simulink model "tanks_model"  (R2014a)
settings: Solver=ode4  StartTime=0.0  StopTime=T  FixedStep=0.001  RelTol=1e-3
values from neighbouring files (symbols this model uses):
  a = 31    [tanks_runner.m]
  b = 40    [tanks_runner.m]
  c = 10    [tanks_runner.m]
  C1 = 20    [tanks_runner.m]
  C2 = 20    [tanks_runner.m]
  C3 = 20    [tanks_runner.m]
  h10 = 13    [tanks_runner.m]
  h20 = 13    [tanks_runner.m]
  h30 = 7    [tanks_runner.m]
  h_max = 40    [tanks_runner.m]
  R = 40    [tanks_runner.m]
  u_max = 50    [tanks_runner.m]
  w = 5    [tanks_runner.m]
settings Model: Creator=Lukasz  LastModifiedBy=Lukasz

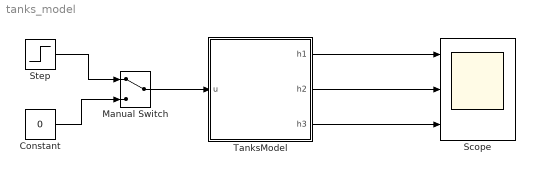
== system tanks_model ==
  Constant : Constant  Value=0
  Manual Switch : ManualSwitch
  Scope : Scope  NumInputPorts=3
      settings: ShowLegends=on  YMin=-0~-5~-5  YMax=40~5~5  SampleInput=on
  Step : Step  Time=0  After=u_max  SampleTime=0
  TanksModel : Subsystem
  wires:
  TanksModel/1(h1) -> Scope/1
  TanksModel/2(h2) -> Scope/2
  TanksModel/3(h3) -> Scope/3
  Manual Switch/1 -> TanksModel/1(u)
  Constant/1 -> Manual Switch/2
  Step/1 -> Manual Switch/1

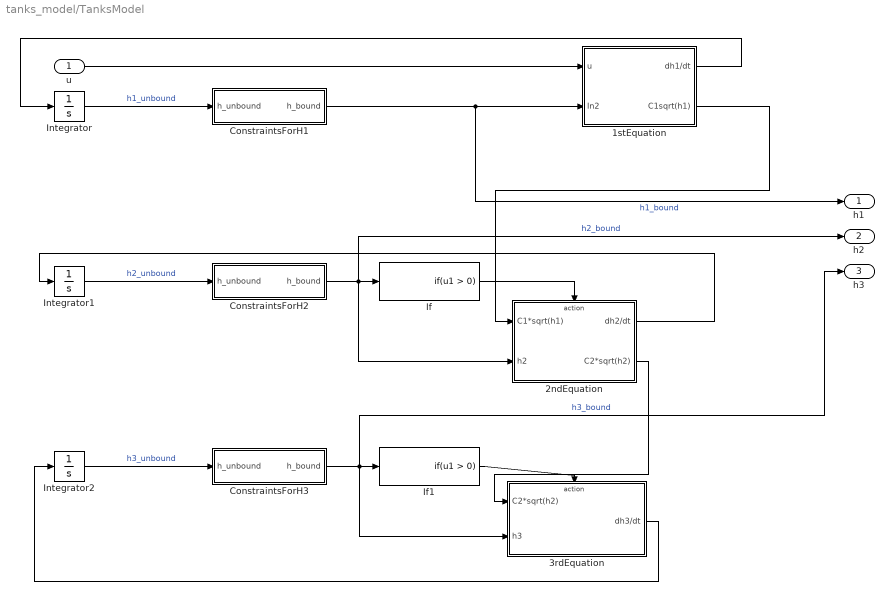
== system tanks_model/TanksModel ==
  u : Inport
  1stEquation : Subsystem
  2ndEquation : Subsystem
  3rdEquation : Subsystem
  ConstraintsForH1 : Subsystem
  ConstraintsForH2 : Subsystem
  ConstraintsForH3 : Subsystem
  If : If  ShowElse=off
  If1 : If  ShowElse=off
  Integrator : Integrator  InitialCondition=h10
  Integrator1 : Integrator  InitialCondition=h20
  Integrator2 : Integrator  InitialCondition=h30
  h1 : Outport
  h2 : Outport  Port=2
  h3 : Outport  Port=3
  wires:
  Integrator1/1 -> ConstraintsForH2/1(h_unbound)  "h2_unbound"
  Integrator2/1 -> ConstraintsForH3/1(h_unbound)  "h3_unbound"
  ConstraintsForH1/1(h_bound) -> h1/1, 1stEquation/2(In2)  "h1_bound"
  Integrator/1 -> ConstraintsForH1/1(h_unbound)  "h1_unbound"
  ConstraintsForH2/1(h_bound) -> If/1, 2ndEquation/2(h2), h2/1  "h2_bound"
  ConstraintsForH3/1(h_bound) -> If1/1, 3rdEquation/2(h3), h3/1  "h3_bound"
  2ndEquation/1(dh2/dt) -> Integrator1/1
  If/1 -> 2ndEquation/Action
  2ndEquation/2(C2*sqrt(h2)) -> 3rdEquation/1(C2*sqrt(h2))
  If1/1 -> 3rdEquation/Action
  3rdEquation/1(dh3/dt) -> Integrator2/1
  u/1 -> 1stEquation/1(u)
  1stEquation/1(dh1/dt) -> Integrator/1
  1stEquation/2(C1sqrt(h1)) -> 2ndEquation/1(C1*sqrt(h1))

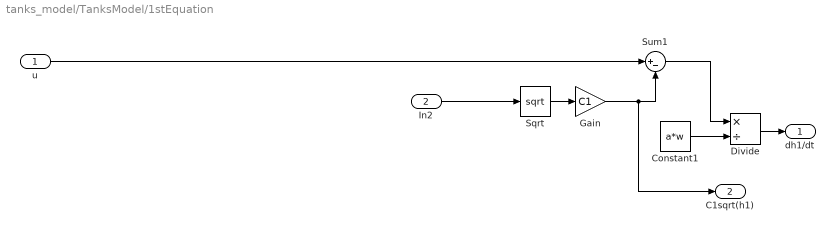
== system tanks_model/TanksModel/1stEquation ==
  u : Inport
  In2 : Inport  Port=2
  Constant1 : Constant  Value=a*w
  Divide : Product  Inputs=*/
  Gain : Gain  Gain=C1
  Sqrt : Sqrt  SaturateOnIntegerOverflow=on
  Sum1 : Sum  Inputs=|+-
  dh1/dt : Outport
  C1sqrt(h1) : Outport  Port=2
  wires:
  In2/1 -> Sqrt/1
  Constant1/1 -> Divide/2
  Divide/1 -> dh1/dt/1
  u/1 -> Sum1/1
  Gain/1 -> C1sqrt(h1)/1, Sum1/2
  Sqrt/1 -> Gain/1
  Sum1/1 -> Divide/1

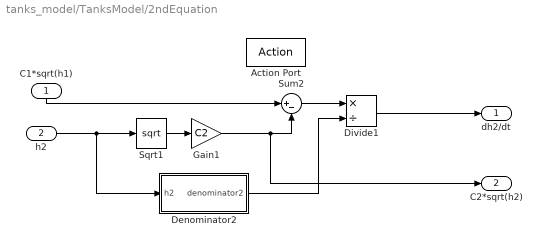
== system tanks_model/TanksModel/2ndEquation ==
  C1*sqrt(h1) : Inport
  h2 : Inport  Port=2
  Action Port : ActionPort  ActionType=then
  Denominator2 : Subsystem
  Divide1 : Product  Inputs=*/
  Gain1 : Gain  Gain=C2
  Sqrt1 : Sqrt  SaturateOnIntegerOverflow=on
  Sum2 : Sum  Inputs=|+-
  dh2/dt : Outport
  C2*sqrt(h2) : Outport  Port=2
  wires:
  Sqrt1/1 -> Gain1/1
  Gain1/1 -> C2*sqrt(h2)/1, Sum2/2
  Denominator2/1(denominator2) -> Divide1/2
  Sum2/1 -> Divide1/1
  Divide1/1 -> dh2/dt/1
  h2/1 -> Denominator2/1(h2), Sqrt1/1
  C1*sqrt(h1)/1 -> Sum2/1

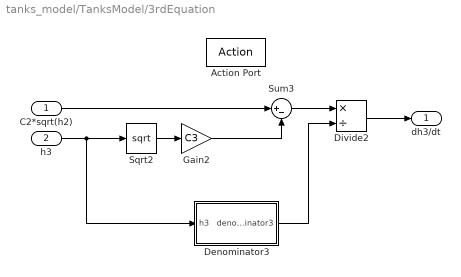
== system tanks_model/TanksModel/3rdEquation ==
  C2*sqrt(h2) : Inport
  h3 : Inport  Port=2
  Action Port : ActionPort  ActionType=then
  Denominator3 : Subsystem
  Divide2 : Product  Inputs=*/
  Gain2 : Gain  Gain=C3
  Sqrt2 : Sqrt  SaturateOnIntegerOverflow=on
  Sum3 : Sum  Inputs=|+-
  dh3/dt : Outport
  wires:
  Sum3/1 -> Divide2/1
  Divide2/1 -> dh3/dt/1
  Sqrt2/1 -> Gain2/1
  Gain2/1 -> Sum3/2
  Denominator3/1(denominator3) -> Divide2/2
  C2*sqrt(h2)/1 -> Sum3/1
  h3/1 -> Denominator3/1(h3), Sqrt2/1

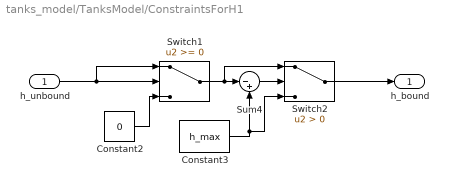
== system tanks_model/TanksModel/ConstraintsForH1 ==
  h_unbound : Inport
  Constant2 : Constant  Value=0
  Constant3 : Constant  Value=h_max
  Sum4 : Sum  Inputs=|-+
  Switch1 : Switch
  Switch2 : Switch  Criteria=u2 > Threshold
  h_bound : Outport
  wires:
  h_unbound/1 -> Switch1/2, Switch1/1
  Constant2/1 -> Switch1/3
  Switch1/1 -> Switch2/1, Sum4/1
  Switch2/1 -> h_bound/1
  Sum4/1 -> Switch2/2
  Constant3/1 -> Sum4/2, Switch2/3

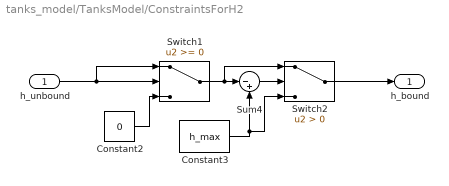
== system tanks_model/TanksModel/ConstraintsForH2 ==
  h_unbound : Inport
  Constant2 : Constant  Value=0
  Constant3 : Constant  Value=h_max
  Sum4 : Sum  Inputs=|-+
  Switch1 : Switch
  Switch2 : Switch  Criteria=u2 > Threshold
  h_bound : Outport
  wires:
  Constant3/1 -> Switch2/3, Sum4/2
  Sum4/1 -> Switch2/2
  Switch2/1 -> h_bound/1
  Switch1/1 -> Sum4/1, Switch2/1
  Constant2/1 -> Switch1/3
  h_unbound/1 -> Switch1/1, Switch1/2

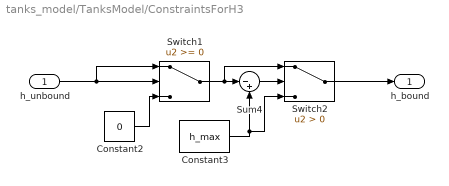
== system tanks_model/TanksModel/ConstraintsForH3 ==
  h_unbound : Inport
  Constant2 : Constant  Value=0
  Constant3 : Constant  Value=h_max
  Sum4 : Sum  Inputs=|-+
  Switch1 : Switch
  Switch2 : Switch  Criteria=u2 > Threshold
  h_bound : Outport
  wires:
  h_unbound/1 -> Switch1/2, Switch1/1
  Constant2/1 -> Switch1/3
  Switch1/1 -> Switch2/1, Sum4/1
  Switch2/1 -> h_bound/1
  Sum4/1 -> Switch2/2
  Constant3/1 -> Sum4/2, Switch2/3

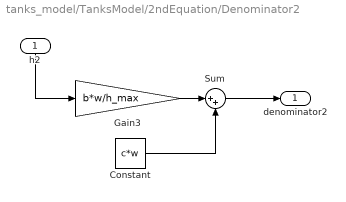
== system tanks_model/TanksModel/2ndEquation/Denominator2 ==
  h2 : Inport
  Constant : Constant  Value=c*w
  Gain3 : Gain  Gain=b*w/h_max
  Sum : Sum  Inputs=|++
  denominator2 : Outport
  wires:
  Sum/1 -> denominator2/1
  Constant/1 -> Sum/2
  h2/1 -> Gain3/1
  Gain3/1 -> Sum/1

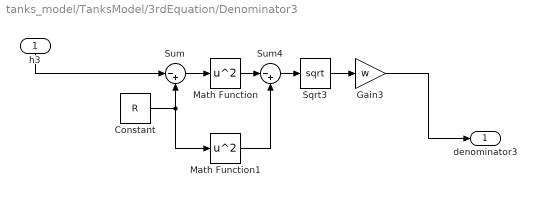
== system tanks_model/TanksModel/3rdEquation/Denominator3 ==
  h3 : Inport
  Constant : Constant  Value=R
  Gain3 : Gain  Gain=w
  Math Function : Math  Operator=square  SaturateOnIntegerOverflow=on
  Math Function1 : Math  Operator=square  SaturateOnIntegerOverflow=on
  Sqrt3 : Sqrt  SaturateOnIntegerOverflow=on
  Sum : Sum  Inputs=|-+
  Sum4 : Sum  Inputs=|-+
  denominator3 : Outport
  wires:
  Sum/1 -> Math Function/1
  Sqrt3/1 -> Gain3/1
  Math Function1/1 -> Sum4/2
  Sum4/1 -> Sqrt3/1
  h3/1 -> Sum/1
  Math Function/1 -> Sum4/1
  Gain3/1 -> denominator3/1
  Constant/1 -> Sum/2, Math Function1/1
